simulink model "inverter_switching_GridFollowing_StudentVersion"  (R2025a)
settings: Solver=ode1be  StartTime=0.0  StopTime=0.2  FixedStep=1e-6  MaxStep=1e-7  RelTol=1e-3
values from neighbouring files (symbols this model uses):
  C_Filter = 300e-6    (= 0.0003)    [parameters_StudentVersion.m]
  kFilterIdq = wnFiltreIdq/WnIdq    (= 1)    [parameters_StudentVersion.m]
  kFilterVdq = wnFiltreVdq/WnVdq    (= 1)    [parameters_StudentVersion.m]
  Kpll2 = 1    [parameters_StudentVersion.m]
  L_Filter = 1e-3    (= 0.001)    [parameters_StudentVersion.m]
  rL_filter = 0.1    [parameters_StudentVersion.m]
  T1 = 10/wcpll    (= 10)    [parameters_StudentVersion.m]
  T2 = 1/(10*wcpll)    (= 0.1)    [parameters_StudentVersion.m]
  T32 = sqrt(2/3)*[1 0; -1/2 sqrt(3)/2; -1/2 -sqrt(3)/2]    [parameters_StudentVersion.m]
  Ts = 1/Fs    (= 5e-05)    [parameters_StudentVersion.m]
  Vdc = 800    [parameters_StudentVersion.m]
  Vrms_Grid = 110    [parameters_StudentVersion.m]
  WnIdq = 12000    [parameters_StudentVersion.m]
  WnVdq = 1200    [parameters_StudentVersion.m]
  wrated = 2*pi*60    (= 376.991118431)    [parameters_StudentVersion.m]
  zeta = 1/sqrt(2)    [parameters_StudentVersion.m]
undefined symbols (not defined in the file or in its folder): DiscIntNeverNeededParam
libraries: nesl_utility x22, ee_lib x16, fl_lib x15, simulink x3
(part 2 of 2)

== system inverter_switching_GridFollowing_StudentVersion/PLL/Vcdq_DG1 ==
  xabc : Inport
  theta_pll : Inport  Port=2
  Demux3 : Demux  Outputs=2
  Fcn : Fcn  Expr=u(1)*cos(u(3))+u(2)*sin(u(3))
  Fcn1 : Fcn  Expr=-u(1)*sin(u(3))+u(2)*cos(u(3))
  Gain11 : Gain  Gain=T32'  Multiplication=Matrix(K*u)
  Mux1 : Mux  Inputs=3
  xd : Outport
  xq : Outport  Port=2
  wires:
  Mux1/1 -> Fcn/1, Fcn1/1
  theta_pll/1 -> Mux1/3
  Demux3/2 -> Mux1/2
  Demux3/1 -> Mux1/1
  Gain11/1 -> Demux3/1
  xabc/1 -> Gain11/1
  Fcn1/1 -> xq/1
  Fcn/1 -> xd/1

== system inverter_switching_GridFollowing_StudentVersion/Transformation/abc to dq0 ==
  xa : Inport
  xb : Inport  Port=2
  xc : Inport  Port=3
  theta : Inport  Port=4
  Fcn : Fcn  Expr=sqrt(2/3)*(u[1]*cos(u[4])+u[2]*cos(u[4]-2*pi/3)+u[3]*cos(u[4]-4*pi/3))
  Fcn1 : Fcn  Expr=sqrt(2/3)*(-u[1]*sin(u[4])-u[2]*sin(u[4]-2*pi/3)-u[3]*sin(u[4]-4*pi/3))
  Fcn2 : Fcn  Expr=sqrt(2/3)*(u[1]+u[2]+u[3])/sqrt(2)
  Mux : Mux
  xd : Outport
  xq : Outport  Port=2
  wires:
  Mux/1 -> Fcn1/1, Fcn/1, Fcn2/1
  Fcn/1 -> xd/1
  Fcn1/1 -> xq/1
  xa/1 -> Mux/1
  xb/1 -> Mux/2
  xc/1 -> Mux/3
  theta/1 -> Mux/4

== system inverter_switching_GridFollowing_StudentVersion/Transformation/abc to dq1 ==
  xa : Inport
  xb : Inport  Port=2
  xc : Inport  Port=3
  theta : Inport  Port=4
  Fcn : Fcn  Expr=sqrt(2/3)*(u[1]*cos(u[4])+u[2]*cos(u[4]-2*pi/3)+u[3]*cos(u[4]-4*pi/3))
  Fcn1 : Fcn  Expr=sqrt(2/3)*(-u[1]*sin(u[4])-u[2]*sin(u[4]-2*pi/3)-u[3]*sin(u[4]-4*pi/3))
  Fcn2 : Fcn  Expr=sqrt(2/3)*(u[1]+u[2]+u[3])/sqrt(2)
  Mux : Mux
  xd : Outport
  xq : Outport  Port=2
  wires:
  theta/1 -> Mux/4
  xc/1 -> Mux/3
  xb/1 -> Mux/2
  xa/1 -> Mux/1
  Fcn1/1 -> xq/1
  Fcn/1 -> xd/1
  Mux/1 -> Fcn2/1, Fcn/1, Fcn1/1

== system inverter_switching_GridFollowing_StudentVersion/Transformation/abc to dq2 ==
  xa : Inport
  xb : Inport  Port=2
  xc : Inport  Port=3
  theta : Inport  Port=4
  Fcn : Fcn  Expr=sqrt(2/3)*(u[1]*cos(u[4])+u[2]*cos(u[4]-2*pi/3)+u[3]*cos(u[4]-4*pi/3))
  Fcn1 : Fcn  Expr=sqrt(2/3)*(-u[1]*sin(u[4])-u[2]*sin(u[4]-2*pi/3)-u[3]*sin(u[4]-4*pi/3))
  Fcn2 : Fcn  Expr=sqrt(2/3)*(u[1]+u[2]+u[3])/sqrt(2)
  Mux : Mux
  xd : Outport
  xq : Outport  Port=2
  wires:
  theta/1 -> Mux/4
  xc/1 -> Mux/3
  xb/1 -> Mux/2
  xa/1 -> Mux/1
  Fcn1/1 -> xq/1
  Fcn/1 -> xd/1
  Mux/1 -> Fcn2/1, Fcn/1, Fcn1/1

== system inverter_switching_GridFollowing_StudentVersion/Transformation/abc to dq8 ==
  xabc : Inport
  theta : Inport  Port=2
  Demux : Demux  Outputs=3
  Fcn : Fcn  Expr=sqrt(2/3)*(u[1]*cos(u[4])+u[2]*cos(u[4]-2*pi/3)+u[3]*cos(u[4]-4*pi/3))
  Fcn1 : Fcn  Expr=sqrt(2/3)*(-u[1]*sin(u[4])-u[2]*sin(u[4]-2*pi/3)-u[3]*sin(u[4]-4*pi/3))
  Fcn2 : Fcn  Expr=sqrt(2/3)*(u[1]+u[2]+u[3])/sqrt(2)
  Mux : Mux
  xd : Outport
  xq : Outport  Port=2
  wires:
  theta/1 -> Mux/4
  Fcn1/1 -> xq/1
  Fcn/1 -> xd/1
  Mux/1 -> Fcn2/1, Fcn/1, Fcn1/1
  Demux/1 -> Mux/1
  Demux/2 -> Mux/2
  Demux/3 -> Mux/3
  xabc/1 -> Demux/1

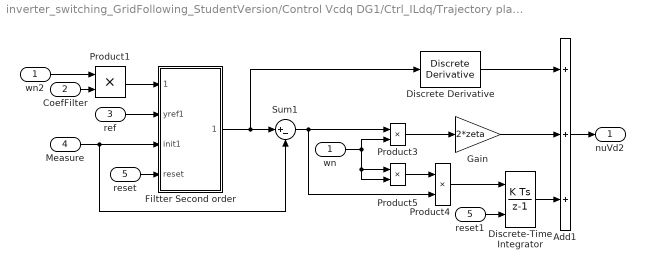
== system inverter_switching_GridFollowing_StudentVersion/Control Vcdq DG1/Ctrl_ILdq/Trajectory planning and Control 1 ==
  wn : Inport
  CoefFilter : Inport  Port=2
  ref : Inport  Port=3
  Measure : Inport  Port=4
  reset : Inport  Port=5
  Add1 : Sum  Inputs=+++
  Discrete Derivative : simulink/Discrete/Discrete Derivative  gainval=1.0  ICPrevScaledInput=0.0  OutMin=[]  OutMax=[]  OutDataType=fixdt(1, 16)  OutScaling=2^-10  DoSatur=off
  Discrete-Time Integrator : DiscreteIntegrator  ExternalReset=level  SampleTime=-1  LimitOutput=on  UpperSaturationLimit=IntegIdLimitPos  LowerSaturationLimit=IntegIdLimitNeg  ICPrevOutput=DiscIntNeverNeededParam  ICPrevScaledInput=DiscIntNeverNeededParam
  Filtter Second order : Subsystem
  Gain : Gain  Gain=2*zeta
  Product{1,3..5} (4 alike) : Product
  Sum1 : Sum  Inputs=|+-
  reset1 : InportShadow  Port=5
  wn2 : InportShadow
  nuVd2 : Outport
  wires:
  Discrete-Time Integrator/1 -> Add1/3
  reset1/1 -> Discrete-Time Integrator/2
  reset/1 -> Filtter Second order/4(reset)
  Sum1/1 -> Product4/2, Product3/1
  Product4/1 -> Discrete-Time Integrator/1
  Product5/1 -> Product4/1
  wn/1 -> Product5/2, Product5/1, Product3/2
  Product3/1 -> Gain/1
  Gain/1 -> Add1/2
  Filtter Second order/1(yref_filtre 1) -> Discrete Derivative/1, Sum1/1
  Product1/1 -> Filtter Second order/1(wfilter2)
  wn2/1 -> Product1/1
  ref/1 -> Filtter Second order/2(yref1)
  Measure/1 -> Sum1/2, Filtter Second order/3(init1)
  CoefFilter/1 -> Product1/2
  Add1/1 -> nuVd2/1
  Discrete Derivative/1 -> Add1/1

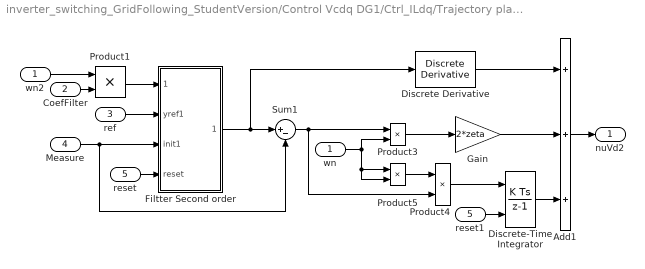
== system inverter_switching_GridFollowing_StudentVersion/Control Vcdq DG1/Ctrl_ILdq/Trajectory planning and Control 2 ==
  wn : Inport
  CoefFilter : Inport  Port=2
  ref : Inport  Port=3
  Measure : Inport  Port=4
  reset : Inport  Port=5
  Add1 : Sum  Inputs=+++
  Discrete Derivative : simulink/Discrete/Discrete Derivative  gainval=1.0  ICPrevScaledInput=0.0  OutMin=[]  OutMax=[]  OutDataType=fixdt(1, 16)  OutScaling=2^-10  DoSatur=off
  Discrete-Time Integrator : DiscreteIntegrator  ExternalReset=level  SampleTime=-1  LimitOutput=on  UpperSaturationLimit=IntegIqLimitPos  LowerSaturationLimit=IntegIqLimitNeg  ICPrevOutput=DiscIntNeverNeededParam  ICPrevScaledInput=DiscIntNeverNeededParam
  Filtter Second order : Subsystem
  Gain : Gain  Gain=2*zeta
  Product{1,3..5} (4 alike) : Product
  Sum1 : Sum  Inputs=|+-
  reset1 : InportShadow  Port=5
  wn2 : InportShadow
  nuVd2 : Outport
  wires:
  Add1/1 -> nuVd2/1
  CoefFilter/1 -> Product1/2
  Measure/1 -> Filtter Second order/3(init1), Sum1/2
  ref/1 -> Filtter Second order/2(yref1)
  wn2/1 -> Product1/1
  Product1/1 -> Filtter Second order/1(wfilter2)
  Filtter Second order/1(yref_filtre 1) -> Discrete Derivative/1, Sum1/1
  Gain/1 -> Add1/2
  Product3/1 -> Gain/1
  wn/1 -> Product3/2, Product5/1, Product5/2
  Product5/1 -> Product4/1
  Product4/1 -> Discrete-Time Integrator/1
  Sum1/1 -> Product3/1, Product4/2
  reset/1 -> Filtter Second order/4(reset)
  reset1/1 -> Discrete-Time Integrator/2
  Discrete-Time Integrator/1 -> Add1/3
  Discrete Derivative/1 -> Add1/1

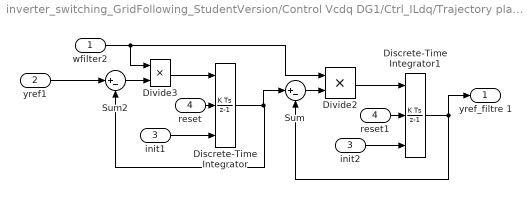
== system inverter_switching_GridFollowing_StudentVersion/Control Vcdq DG1/Ctrl_ILdq/Trajectory planning and Control 1/Filtter Second order ==
  wfilter2 : Inport
  yref1 : Inport  Port=2
  init1 : Inport  Port=3
  reset : Inport  Port=4
  Discrete-Time Integrator : DiscreteIntegrator  ExternalReset=level  InitialConditionSource=external  SampleTime=-1  ICPrevOutput=DiscIntNeverNeededParam  ICPrevScaledInput=DiscIntNeverNeededParam
  Discrete-Time Integrator1 : DiscreteIntegrator  ExternalReset=level  InitialConditionSource=external  SampleTime=-1  ICPrevOutput=DiscIntNeverNeededParam  ICPrevScaledInput=DiscIntNeverNeededParam
  Divide2 : Product  Inputs=**
  Divide3 : Product  Inputs=**
  Sum : Sum  Inputs=|+-
  Sum2 : Sum  Inputs=|+-
  init2 : InportShadow  Port=3
  reset1 : InportShadow  Port=4
  yref_filtre 1 : Outport
  wires:
  reset1/1 -> Discrete-Time Integrator1/2
  reset/1 -> Discrete-Time Integrator/2
  init2/1 -> Discrete-Time Integrator1/3
  Sum2/1 -> Divide3/2
  Discrete-Time Integrator1/1 -> yref_filtre 1/1, Sum/2
  yref1/1 -> Sum2/1
  Sum/1 -> Divide2/2
  Divide3/1 -> Discrete-Time Integrator/1
  Discrete-Time Integrator/1 -> Sum/1, Sum2/2
  init1/1 -> Discrete-Time Integrator/3
  wfilter2/1 -> Divide3/1, Divide2/1
  Divide2/1 -> Discrete-Time Integrator1/1

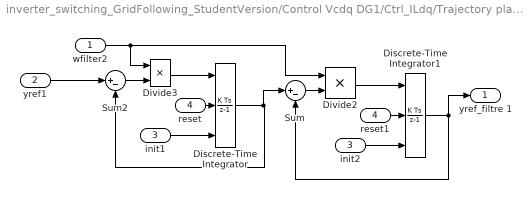
== system inverter_switching_GridFollowing_StudentVersion/Control Vcdq DG1/Ctrl_ILdq/Trajectory planning and Control 2/Filtter Second order ==
  wfilter2 : Inport
  yref1 : Inport  Port=2
  init1 : Inport  Port=3
  reset : Inport  Port=4
  Discrete-Time Integrator : DiscreteIntegrator  ExternalReset=level  InitialConditionSource=external  SampleTime=-1  ICPrevOutput=DiscIntNeverNeededParam  ICPrevScaledInput=DiscIntNeverNeededParam
  Discrete-Time Integrator1 : DiscreteIntegrator  ExternalReset=level  InitialConditionSource=external  SampleTime=-1  ICPrevOutput=DiscIntNeverNeededParam  ICPrevScaledInput=DiscIntNeverNeededParam
  Divide2 : Product  Inputs=**
  Divide3 : Product  Inputs=**
  Sum : Sum  Inputs=|+-
  Sum2 : Sum  Inputs=|+-
  init2 : InportShadow  Port=3
  reset1 : InportShadow  Port=4
  yref_filtre 1 : Outport
  wires:
  Divide2/1 -> Discrete-Time Integrator1/1
  wfilter2/1 -> Divide2/1, Divide3/1
  init1/1 -> Discrete-Time Integrator/3
  Discrete-Time Integrator/1 -> Sum2/2, Sum/1
  Divide3/1 -> Discrete-Time Integrator/1
  Sum/1 -> Divide2/2
  yref1/1 -> Sum2/1
  Discrete-Time Integrator1/1 -> Sum/2, yref_filtre 1/1
  Sum2/1 -> Divide3/2
  init2/1 -> Discrete-Time Integrator1/3
  reset/1 -> Discrete-Time Integrator/2
  reset1/1 -> Discrete-Time Integrator1/2
